simulink model "PoliArd_LQR_Kalman_2015a"  (R2015a)
settings: Solver=ode3  StartTime=0.0  StopTime=inf  FixedStep=0.001  RelTol=1e-3
values from neighbouring files (symbols this model uses):
  A_obs = A    [Main_PoliArd_LQR_Kalman.m]
  b = 0.0245    [Main_Circle_traj_generation.m]    (also in Main_Manual_trajectory_generation.m; Main_PoliArd_LQR_Kalman.m)
  Bx_obs = [Bx Kx_obs]    [Main_PoliArd_LQR_Kalman.m]
  By_obs = [By Ky_obs]    [Main_PoliArd_LQR_Kalman.m]
  C = [1 0]    [Main_PoliArd_LQR_Kalman.m]    (also in dfdu.m = data)
  C_obs = eye(2)    [Main_PoliArd_LQR_Kalman.m]
  D_obs = zeros(2)    [Main_PoliArd_LQR_Kalman.m]
  ICx_obs = [0 0]'    [Main_PoliArd_LQR_Kalman.m]
  ICy_obs = [0 0]'    [Main_PoliArd_LQR_Kalman.m]
undefined symbols (not defined in the file or in its folder): cx, cy
libraries: PoliArd x6, simulink_extras x2
settings Model: CovHtmlReporting=off  ExtModeTrigDuration=2  Creator=User  LastModifiedBy=User
settings OptimizationCC: LifeSpan=1
settings DebuggingCC: UnderspecifiedInitializationDetection=Classic  MergeDetectMultiDrivingBlocksExec=none
settings HardwareCC: ProdLargestAtomicInteger=Long  ProdLargestAtomicFloat=Double  ProdEndianess=LittleEndian  ProdHWDeviceType=ARM Compatible->ARM Cortex
settings RTWCC: SystemTargetFile=realtime.tlc  GenerateMakefile=off  TemplateMakefile=realtime.tmf  Description=Run on Target Hardware  RTWVerbose=off
settings ERTTargetCC: CombineOutputUpdateFcns=off  ExtModeTransport=3  ExtModeMexFile=ext_serial_win32_comm_rtt  ExtModeMexArgs=0 1 9600  InlinedParameterPlacement=Hierarchical  ERTSrcFileBannerTemplate=realtime_code_template.cgt  ERTHdrFileBannerTemplate=realtime_code_template.cgt  ERTDataSrcFileTemplate=realtime_code_template.cgt  ERTDataHdrFileTemplate=realtime_code_template.cgt  ERTCustomFileTemplate=realtime_file_process.tlc

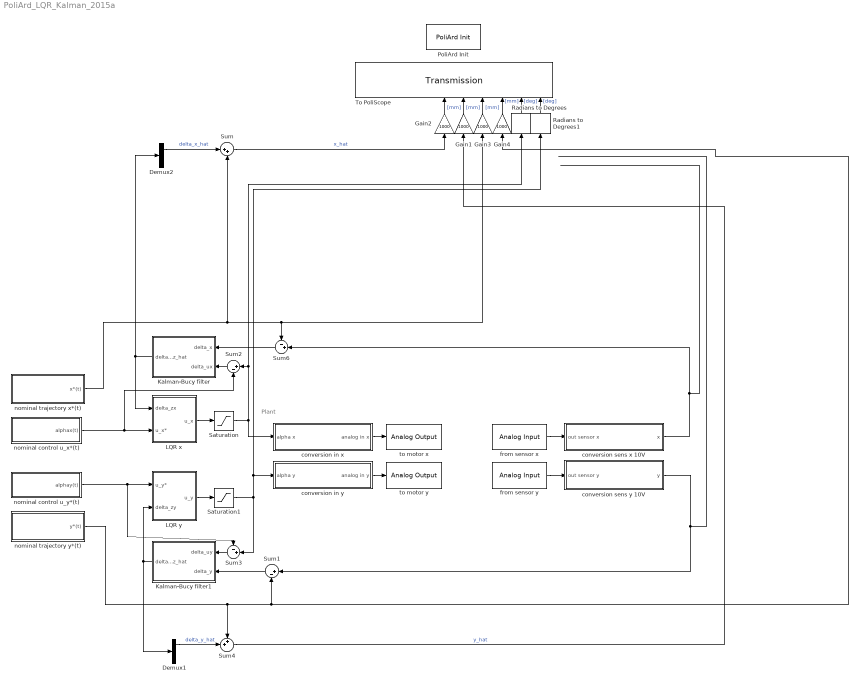
== system PoliArd_LQR_Kalman_2015a ==
  note: Plant
  Demux1 : Demux  Outputs=2
  Demux2 : Demux  Outputs=2
  Gain{1..4} (4 alike) : Gain  Gain=1000
  Kalman-Bucy filter : Subsystem
  Kalman-Bucy filter1 : Subsystem
  LQR x : Subsystem
  LQR y : Subsystem
  PoliArd Init : PoliArd/PoliArd Init
  Radians to Degrees : simulink_extras/Transformations/Radians to Degrees
  Radians to Degrees1 : simulink_extras/Transformations/Radians to Degrees
  Saturation : Saturate  UpperLimit=deg2rad(75)  LowerLimit=deg2rad(-75)
  Saturation1 : Saturate  UpperLimit=deg2rad(75)  LowerLimit=deg2rad(-75)
  Sum : Sum  Inputs=|++
  Sum1 : Sum  Inputs=|+-
  Sum2 : Sum  Inputs=|+-
  Sum3 : Sum  Inputs=-+|
  Sum4 : Sum  Inputs=++|
  Sum6 : Sum  Inputs=-+|
  To PoliScope : PoliArd/Transmission  sample_freq=1000  sig_to_send=6
  conversion in x : Subsystem
  conversion in y : Subsystem
  conversion sens x 10V : Subsystem
  conversion sens y 10V : Subsystem
  from sensor x : PoliArd/Analog Input  AIpin_mask=4  AIsample=-1
  from sensor y : PoliArd/Analog Input  AIpin_mask=3  AIsample=-1
  nominal control u_x*(t) : Subsystem
  nominal control u_y*(t) : Subsystem
  nominal trajectory x*(t) : Subsystem
  nominal trajectory y*(t) : Subsystem
  to motor x : PoliArd/Analog Output  DAC_pin_mask=1
  to motor y : PoliArd/Analog Output  DAC_pin_mask=2
  wires:
  from sensor x/1 -> conversion sens x 10V/1(out sensor x)
  from sensor y/1 -> conversion sens y 10V/1(out sensor y)
  conversion in x/1(analog in x) -> to motor x/1
  Gain2/1 -> To PoliScope/5  "[mm]"
  Gain1/1 -> To PoliScope/6  "[mm]"
  Radians to Degrees/1 -> To PoliScope/9  "[deg]"
  conversion in y/1(analog in y) -> to motor y/1
  Saturation/1 -> conversion in x/1(alpha x), Sum2/1, Radians to Degrees/1
  Saturation1/1 -> Radians to Degrees1/1, conversion in y/1(alpha y), Sum3/2
  Gain3/1 -> To PoliScope/7  "[mm]"
  Gain4/1 -> To PoliScope/8  "[mm]"
  Radians to Degrees1/1 -> To PoliScope/10  "[deg]"
  LQR x/1(u_x) -> Saturation/1
  LQR y/1(u_y) -> Saturation1/1
  Kalman-Bucy filter/1(delta_z_hat) -> Demux2/1, LQR x/1(delta_zx)
  Kalman-Bucy filter1/1(delta_z_hat) -> LQR y/2(delta_zy), Demux1/1
  nominal control u_x*(t)/1(alphax(t)) -> Sum2/2, LQR x/2(u_x*)
  nominal control u_y*(t)/1(alphay(t)) -> Sum3/1, LQR y/1(u_y*)
  conversion sens x 10V/1(x) -> Sum6/2
  Sum/1 -> Gain2/1  "x_hat"
  Sum4/1 -> Gain1/1  "y_hat"
  conversion sens y 10V/1(y) -> Sum1/1
  nominal trajectory x*(t)/1(x*(t)) -> Sum/2, Gain3/1, Sum6/1
  Sum6/1 -> Kalman-Bucy filter/1(delta_x)
  nominal trajectory y*(t)/1(y*(t)) -> Sum1/2, Gain4/1, Sum4/1
  Sum1/1 -> Kalman-Bucy filter1/2(delta_y)
  Sum3/1 -> Kalman-Bucy filter1/1(delta_uy)
  Sum2/1 -> Kalman-Bucy filter/2(delta_ux)
  Demux2/1 -> Sum/1  "delta_x_hat"
  Demux1/1 -> Sum4/2  "delta_y_hat"

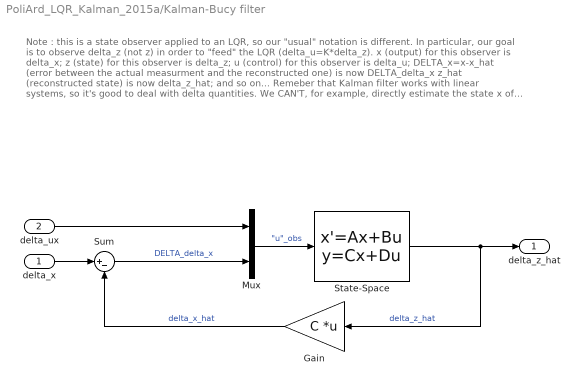
== system PoliArd_LQR_Kalman_2015a/Kalman-Bucy filter ==
  note: Note : this is a state observer applied to an LQR, so our "usual" notation is different. In particular, our goal is to observe delta_z (not z) in order to "feed" the LQR (delta_u=K*delta_z).
      |
      | x (output) for this observer is delta_x;
      | z (state) for this observer is delta_z;
      | u (control) for this observer is delta_u;
      | DELTA_x=x-x_hat (error between the actual measurment and the reconstructed one) is now DELTA_delta_x
      | z_hat (reconstructed state) is now delta_z_hat;
      | and so on...
      |
      | Remeber that Kalman filter works with linear systems, so it's good to deal with delta quantities. We CAN'T, for example, directly estimate the state x of the nonlinear system (we need a nonlinear observer for that, for exemple an extension of Kalman filter).
  delta_x : Inport
  delta_ux : Inport  Port=2
  Gain : Gain  Gain=C  Multiplication=Matrix(K*u) (u vector)
  Mux : Mux  Inputs=2
  State-Space : StateSpace  A=A_obs  B=Bx_obs  C=C_obs  D=D_obs  X0=ICx_obs
  Sum : Sum  Inputs=|+-
  delta_z_hat : Outport
  wires:
  State-Space/1 -> delta_z_hat/1, Gain/1  "delta_z_hat"
  delta_ux/1 -> Mux/1
  Mux/1 -> State-Space/1  "\"u\"_obs"
  Sum/1 -> Mux/2  "DELTA_delta_x"
  delta_x/1 -> Sum/1
  Gain/1 -> Sum/2  "delta_x_hat"

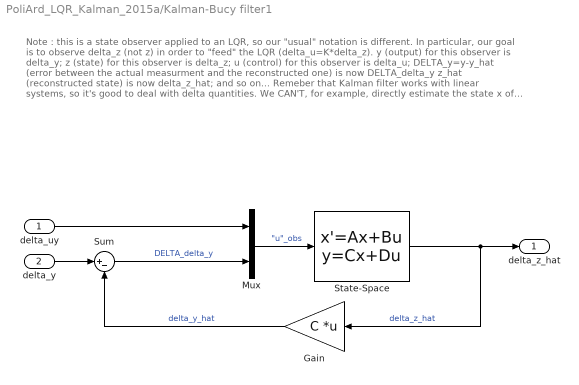
== system PoliArd_LQR_Kalman_2015a/Kalman-Bucy filter1 ==
  note: Note : this is a state observer applied to an LQR, so our "usual" notation is different. In particular, our goal is to observe delta_z (not z) in order to "feed" the LQR (delta_u=K*delta_z).
      |
      | y (output) for this observer is delta_y;
      | z (state) for this observer is delta_z;
      | u (control) for this observer is delta_u;
      | DELTA_y=y-y_hat (error between the actual measurment and the reconstructed one) is now DELTA_delta_y
      | z_hat (reconstructed state) is now delta_z_hat;
      | and so on...
      |
      | Remeber that Kalman filter works with linear systems, so it's good to deal with delta quantities. We CAN'T, for example, directly estimate the state x of the nonlinear system (we need a nonlinear observer for that, for exemple an extension of Kalman filter).
  delta_uy : Inport
  delta_y : Inport  Port=2
  Gain : Gain  Gain=C  Multiplication=Matrix(K*u) (u vector)
  Mux : Mux  Inputs=2
  State-Space : StateSpace  A=A_obs  B=By_obs  C=C_obs  D=D_obs  X0=ICy_obs
  Sum : Sum  Inputs=|+-
  delta_z_hat : Outport
  wires:
  Gain/1 -> Sum/2  "delta_y_hat"
  delta_y/1 -> Sum/1
  Sum/1 -> Mux/2  "DELTA_delta_y"
  Mux/1 -> State-Space/1  "\"u\"_obs"
  delta_uy/1 -> Mux/1
  State-Space/1 -> Gain/1, delta_z_hat/1  "delta_z_hat"

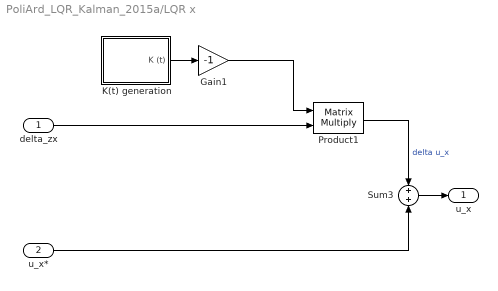
== system PoliArd_LQR_Kalman_2015a/LQR x ==
  delta_zx : Inport
  u_x* : Inport  Port=2
  Gain1 : Gain  Gain=-1
  K(t) generation : Subsystem
  Product1 : Product  Multiplication=Matrix(*)
  Sum3 : Sum
  u_x : Outport
  wires:
  Sum3/1 -> u_x/1
  delta_zx/1 -> Product1/2
  u_x*/1 -> Sum3/2
  K(t) generation/1(K (t)) -> Gain1/1
  Gain1/1 -> Product1/1
  Product1/1 -> Sum3/1  "delta u_x"

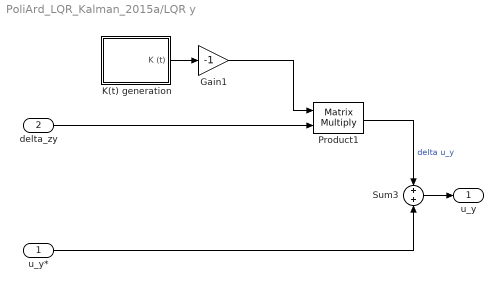
== system PoliArd_LQR_Kalman_2015a/LQR y ==
  u_y* : Inport
  delta_zy : Inport  Port=2
  Gain1 : Gain  Gain=-1
  K(t) generation : Subsystem
  Product1 : Product  Multiplication=Matrix(*)
  Sum3 : Sum
  u_y : Outport
  wires:
  delta_zy/1 -> Product1/2
  Sum3/1 -> u_y/1
  Product1/1 -> Sum3/1  "delta u_y"
  u_y*/1 -> Sum3/2
  Gain1/1 -> Product1/1
  K(t) generation/1(K (t)) -> Gain1/1

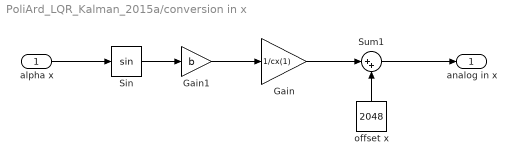
== system PoliArd_LQR_Kalman_2015a/conversion in x ==
  alpha x : Inport
  Gain : Gain  Gain=1/cx(1)
  Gain1 : Gain  Gain=b
  Sin : Trigonometry
  Sum1 : Sum  Inputs=|++
  offset x : Constant  Value=2048
  analog in x : Outport
  wires:
  alpha x/1 -> Sin/1
  offset x/1 -> Sum1/2
  Sum1/1 -> analog in x/1
  Gain/1 -> Sum1/1
  Gain1/1 -> Gain/1
  Sin/1 -> Gain1/1

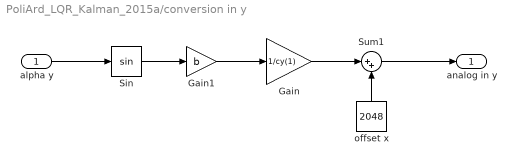
== system PoliArd_LQR_Kalman_2015a/conversion in y ==
  alpha y : Inport
  Gain : Gain  Gain=1/cy(1)
  Gain1 : Gain  Gain=b
  Sin : Trigonometry
  Sum1 : Sum  Inputs=|++
  offset x : Constant  Value=2048
  analog in y : Outport
  wires:
  Sin/1 -> Gain1/1
  Gain1/1 -> Gain/1
  Gain/1 -> Sum1/1
  Sum1/1 -> analog in y/1
  offset x/1 -> Sum1/2
  alpha y/1 -> Sin/1

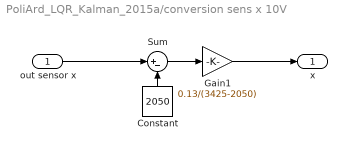
== system PoliArd_LQR_Kalman_2015a/conversion sens x 10V ==
  out sensor x : Inport
  Constant : Constant  Value=2050
  Gain1 : Gain  Gain=0.13/(3425-2050)
  Sum : Sum  Inputs=|+-
  x : Outport
  wires:
  Gain1/1 -> x/1
  out sensor x/1 -> Sum/1
  Sum/1 -> Gain1/1
  Constant/1 -> Sum/2

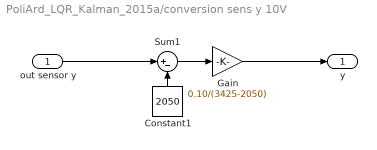
== system PoliArd_LQR_Kalman_2015a/conversion sens y 10V ==
  out sensor y : Inport
  Constant1 : Constant  Value=2050
  Gain : Gain  Gain=0.10/(3425-2050)
  Sum1 : Sum  Inputs=|+-
  y : Outport
  wires:
  Gain/1 -> y/1
  Constant1/1 -> Sum1/2
  Sum1/1 -> Gain/1
  out sensor y/1 -> Sum1/1

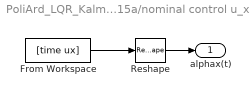
== system PoliArd_LQR_Kalman_2015a/nominal control u_x*(t) ==
  From Workspace : FromWorkspace  VariableName=[time ux]  SampleTime=0  OutputAfterFinalValue=Holding final value
  Reshape : Reshape  OutputDimensionality=Column vector (2-D)
  alphax(t) : Outport
  wires:
  Reshape/1 -> alphax(t)/1
  From Workspace/1 -> Reshape/1

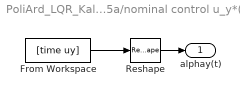
== system PoliArd_LQR_Kalman_2015a/nominal control u_y*(t) ==
  From Workspace : FromWorkspace  VariableName=[time uy]  SampleTime=0  OutputAfterFinalValue=Holding final value
  Reshape : Reshape  OutputDimensionality=Column vector (2-D)
  alphay(t) : Outport
  wires:
  Reshape/1 -> alphay(t)/1
  From Workspace/1 -> Reshape/1

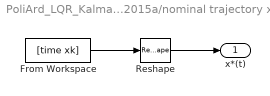
== system PoliArd_LQR_Kalman_2015a/nominal trajectory x*(t) ==
  From Workspace : FromWorkspace  VariableName=[time xk]  SampleTime=0  OutputAfterFinalValue=Holding final value
  Reshape : Reshape  OutputDimensionality=Column vector (2-D)
  x*(t) : Outport
  wires:
  Reshape/1 -> x*(t)/1
  From Workspace/1 -> Reshape/1

== system PoliArd_LQR_Kalman_2015a/nominal trajectory y*(t) ==
  From Workspace : FromWorkspace  VariableName=[time yk]  SampleTime=0  OutputAfterFinalValue=Holding final value
  Reshape : Reshape  OutputDimensionality=Column vector (2-D)
  y*(t) : Outport
  wires:
  Reshape/1 -> y*(t)/1
  From Workspace/1 -> Reshape/1

== system PoliArd_LQR_Kalman_2015a/LQR x/K(t) generation ==
  From Workspace : FromWorkspace  VariableName=[time Kx_lqr]  SampleTime=0  OutputAfterFinalValue=Holding final value
  Reshape : Reshape  OutputDimensionality=Row vector (2-D)
  K (t) : Outport
  wires:
  Reshape/1 -> K (t)/1
  From Workspace/1 -> Reshape/1

== system PoliArd_LQR_Kalman_2015a/LQR y/K(t) generation ==
  From Workspace : FromWorkspace  VariableName=[time Ky_lqr]  SampleTime=0  OutputAfterFinalValue=Holding final value
  Reshape : Reshape  OutputDimensionality=Row vector (2-D)
  K (t) : Outport
  wires:
  Reshape/1 -> K (t)/1
  From Workspace/1 -> Reshape/1
